simulink model "KBM_sim"  (R2020b)
settings: Solver=FixedStepAuto  StartTime=0.0  StopTime=100  FixedStep=dt  RelTol=1e-3
values from neighbouring files (symbols this model uses):
  B = 5    [impedance_evaluation_sim.m]
  dt = 1e-3    (= 0.001)    [impedance_evaluation_sim.m]
  ext_signal = 1    [impedance_evaluation_sim.m]
  K = 200    [impedance_evaluation_sim.m]
  M = 0.1    [impedance_evaluation_sim.m]
  pert_duration = 0.060/dt    (= 60)    [impedance_evaluation_sim.m]
  pert_mag = 1    [impedance_evaluation_sim.m]
  pert_space = ceil(3.3/dt)    [impedance_evaluation_sim.m]
settings Model: Creator=fortineau_vin  LastModifiedBy=fortineau_vin

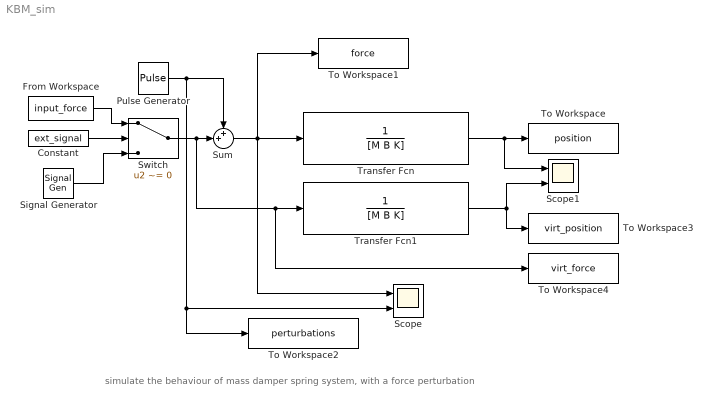
== system KBM_sim ==
  note: simulate the behaviour of mass damper spring system, with a force perturbation
  Constant : Constant  Value=ext_signal
  From Workspace : FromWorkspace  VariableName=input_force  SampleTime=dt
  Pulse Generator : DiscretePulseGenerator  Amplitude=pert_mag  Period=pert_space  PulseWidth=pert_duration  PhaseDelay=5000  SampleTime=dt
  Scope : Scope  NumInputPorts=2
  Scope1 : Scope  NumInputPorts=2
  Signal Generator : SignalGenerator  Amplitude=5
  Sum : Sum  Inputs=++|
  Switch : Switch  Criteria=u2 ~= 0
  To Workspace : ToWorkspace  VariableName=position  SaveFormat=Timeseries  SampleTime=-1
  To Workspace1 : ToWorkspace  VariableName=force  SaveFormat=Timeseries  SampleTime=-1
  To Workspace2 : ToWorkspace  VariableName=perturbations  SaveFormat=Timeseries  SampleTime=-1
  To Workspace3 : ToWorkspace  VariableName=virt_position  SaveFormat=Timeseries  SampleTime=-1
  To Workspace4 : ToWorkspace  VariableName=virt_force  SaveFormat=Timeseries  SampleTime=-1
  Transfer Fcn : TransferFcn  Denominator=[M B K]
  Transfer Fcn1 : TransferFcn  Denominator=[M B K]
  wires:
  Sum/1 -> Scope/1, To Workspace1/1, Transfer Fcn/1
  Transfer Fcn/1 -> Scope1/1, To Workspace/1
  Pulse Generator/1 -> To Workspace2/1, Scope/2, Sum/1
  Switch/1 -> To Workspace4/1, Transfer Fcn1/1, Sum/2
  Constant/1 -> Switch/2
  From Workspace/1 -> Switch/1
  Signal Generator/1 -> Switch/3
  Transfer Fcn1/1 -> To Workspace3/1, Scope1/2
